simulink model "ssm_airframe_thrustvectored_test"  (R2022a)
settings: Solver=ode45  StartTime=0.0  StopTime=SimTime  RelTol=1e-3  AbsTol=1e-6
PreLoadFcn:
  | airframe_init
StopFcn:
  | airframe_plot
values from neighbouring files (symbols this model uses):
  ArmLength = 0.820 + 1.540    (= 2.36)    [airframe_init.m]
  boosting_time = 5    [airframe_init.m]
  thrust_magnitude = 78*1e+3    (= 78000)    [airframe_init.m]
undefined symbols (not defined in the file or in its folder): sigbuilder_block
libraries: shared6dof x1, simulink x1, simulink_extras x1
settings Model: Creator=amani  LastModifiedBy=amani

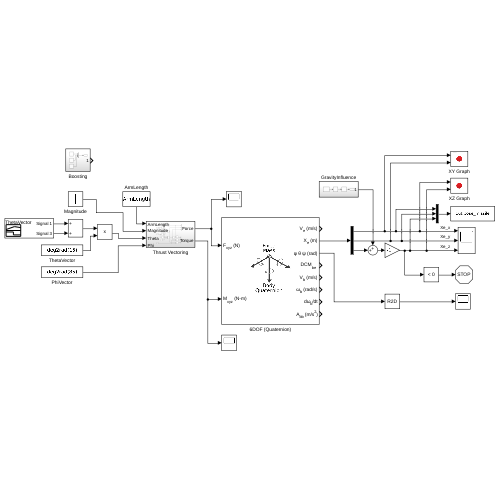
[thumbnail: Simulink's stored preview of the top-level diagram]
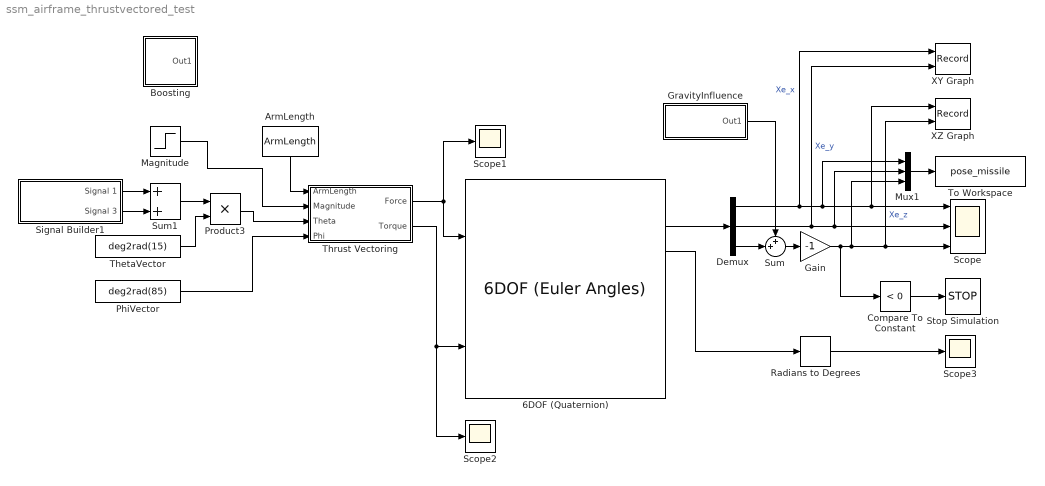
== system ssm_airframe_thrustvectored_test ==
  6DOF (Quaternion) : shared6dof/6DOF (Euler Angles)  units=Metric (MKS)  mtype=Fixed  rep=Quaternion  xme_0=pose_ini  Vm_0=vel_ini  eul_0=rot_ini  pm_0=rotvel_ini  mass_0=mass  mass_e=0.5  mass_f=2.0  inertia=inertia  inertia_e=eye(3)  inertia_f=2*eye(3)  k_quat=1.0  vre_flag=on  abi_flag=off  aMode=0  xme_statename=''  Vm_statename=''  eul_statename=''  quat_statename=''  pm_statename=''  mass_statename=''
      settings: SourceProductBaseCode=AE,PW,DR,MT,VE
  ArmLength : Constant  Value=ArmLength  VectorParams1D=off
  Boosting : Subsystem
  Compare To Constant : simulink/Logic and Bit Operations/Compare To Constant  relop=<  const=0  OutDataTypeStr=boolean
  Demux : Demux  Outputs=3
  Gain : Gain  Gain=-1
  GravityInfluence : Subsystem
  Magnitude : Step  Time=5  Before=thrust_magnitude  After=0  SampleTime=0
  Mux1 : Mux  Inputs=3
  PhiVector : Constant  Value=deg2rad(85)
  Product3 : Product
  Radians to Degrees : simulink_extras/Transformations/Radians to Degrees
  Scope : Scope  NumInputPorts=3
  Scope1 : Scope
  Scope2 : Scope
  Scope3 : Scope
  Signal Builder1 : Subsystem  Tag=STV Subsys  LoadFcn=sigbuilder_block('load');  StartFcn=sigbuilder_block('start');  StopFcn=sigbuilder_block('stop');  ClipboardFcn=sigbuilder_block('clipboard');  mask(Sigbuilder block){tuvar=[0:10]}
      mask help: Simulink:masks:SigbuilderBlock_MD
      mask init:
      | if ~strcmp(get_param(bdroot(gcbh),'SimulationStatus'),'stopped') tuvar = sigbuilder_block('maskInit'); end
      settings: CopyFcn=sigbuilder_block('copy');  DeleteFcn=sigbuilder_block('delete');  ModelCloseFcn=sigbuilder_block('modelClose');  PreSaveFcn=sigbuilder_block('preSave');  PauseFcn=sigbuilder_block('pause');  ContinueFcn=sigbuilder_block('continue');  NameChangeFcn=sigbuilder_block('namechange');  OpenFcn=sigbuilder_block('open',[40.5 0 1399.5 720.75 ]);  CloseFcn=sigbuilder_block('close');
      mask Display: plot(0, 0, 100, 100,[2, 2, 32, 32, 2], [68, 8, 8, 68, 68],[32, 2], [38, 38], [32, 19, 2],[53, 60, 44], [32, 17, 17, 2],[16, 16, 31, 31]);txt = getActiveGroup(gcbh);text(2, 100, txt,'verticalAlignment', 'top');
  Stop Simulation : Stop
  Sum : Sum  Inputs=++|
  Sum1 : Sum
  ThetaVector : Constant  Value=deg2rad(15)
  Thrust Vectoring : Subsystem
  To Workspace : ToWorkspace  VariableName=pose_missile  SaveFormat=Structure With Time  SampleTime=-1
  XY Graph : Record  FileSettingsInternal="{\"entries\":[{\"content\":{\"excelSettings\":{\"content\":{},\"type\":\"Streamout.ExcelSettings\"}},\"type\":\"Streamout.FileSettingStorage\",\"uuid\":\"0ebe5bd2-6dd8-4422-9468-a2e5212a589c\"}],\"packageUris\":[\"http://schema.mathworks.com/mf0/streamout_blocks/R2020a\"],\"version\":\"1.0\"}"  Layout=[1 1]  SignalsInternal="{\"entries\":[{\"content\":{\"signals\":[{\"content\":{\"blockPath\":[\"ssm_airframe_thrustvectored_test/XY Graph\"],\"channel\":[],\"dimensions\":[1],\"domain\":\"ssm_airframe_thrustvectored_test/XY Graph\",\"lineColor\":\"#a2142f\",\"plots\":[1],\"port\":1,\"sid\":[\"\"],\"signalID\":2033,\"signalName\":\"Xe_x\"},\"type\":\"RecordBlkView.Signal\",\"uuid\":\"929725db-a9ff-4e40-934e-6f60430dcc31\"},{\"content\":{\"blockPath\":[\"ssm_airframe_thrustvectored_test/XY Graph\"],\"channel\":[],\"dimensions\":[1],\"domain\":\"ssm_airframe_thrustvectored_test/XY Graph\",\"lineColor\":\"#139fff\",\"plots\":[1],\"port\":2,\"sid\":[\"\"],\"signalID\":2037,\"signalName\":\"Xe_y\"},\"type\":\"RecordBlkView.Signal\",\"uuid\":\"1de2dc4e-5c32-4d5d-ac98-cd5ddb664dcb\"}]},\"type\":\"RecordBlkView.InputSignals\",\"uuid\":\"a82f1b7b-1438-4de9-aa00-4fe59ea993c8\"}],\"packageUris\":[\"http://schema.mathworks.com/mf0/streamout_blocks/R2020a\"],\"version\":\"1.0\"}"  VisualizationBindings="{\"xyplotplugin\":{\"info\":[{\"series\":[{\"bindingParametersList\":[{\"parameter\":\"X-Axis\",\"signalID\":2033,\"signalName\":\"Xe_x\"},{\"parameter\":\"Y-Axis\",\"signalID\":2037,\"signalName\":\"Xe_y\"}],\"seriesID\":26156}],\"subplotID\":1}]}}"  CompatibilityTag=XY
  XZ Graph : Record  FileSettingsInternal="{\"entries\":[{\"content\":{\"excelSettings\":{\"content\":{},\"type\":\"Streamout.ExcelSettings\"}},\"type\":\"Streamout.FileSettingStorage\",\"uuid\":\"bbd1cac7-7029-4a9d-b9ac-d55883903ed7\"}],\"packageUris\":[\"http://schema.mathworks.com/mf0/streamout_blocks/R2020a\"],\"version\":\"1.0\"}"  Layout=[1 1]  SignalsInternal="{\"entries\":[{\"content\":{\"signals\":[{\"content\":{\"blockPath\":[\"ssm_airframe_thrustvectored_test/XZ Graph\"],\"channel\":[],\"dimensions\":[1],\"domain\":\"ssm_airframe_thrustvectored_test/XZ Graph\",\"lineColor\":\"#a2142f\",\"plots\":[1],\"port\":1,\"sid\":[\"\"],\"signalID\":2041,\"signalName\":\"Xe_x\"},\"type\":\"RecordBlkView.Signal\",\"uuid\":\"0a9b8eae-95df-4890-bdce-3116e9e64470\"},{\"content\":{\"blockPath\":[\"ssm_airframe_thrustvectored_test/XZ Graph\"],\"channel\":[],\"dimensions\":[1],\"domain\":\"ssm_airframe_thrustvectored_test/XZ Graph\",\"lineColor\":\"#139fff\",\"plots\":[1],\"port\":2,\"sid\":[\"\"],\"signalID\":2045,\"signalName\":\"Xe_z\"},\"type\":\"RecordBlkView.Signal\",\"uuid\":\"3959e62f-dd22-4433-954b-9d04f4581c5f\"}]},\"type\":\"RecordBlkView.InputSignals\",\"uuid\":\"aa5ce69c-9ff5-428d-bb5e-9516fd4365a3\"}],\"packageUris\":[\"http://schema.mathworks.com/mf0/streamout_blocks/R2020a\"],\"version\":\"1.0\"}"  VisualizationBindings="{\"xyplotplugin\":{\"info\":[{\"series\":[{\"bindingParametersList\":[{\"parameter\":\"X-Axis\",\"signalID\":2041,\"signalName\":\"Xe_x\"},{\"parameter\":\"Y-Axis\",\"signalID\":2045,\"signalName\":\"Xe_z\"}],\"seriesID\":25179}],\"subplotID\":1}]}}"  CompatibilityTag=XY
  wires:
  6DOF (Quaternion)/2 -> Demux/1
  Gain/1 -> XZ Graph/2, Scope/3, Mux1/3, Compare To Constant/1  "Xe_z"
  Sum/1 -> Gain/1
  Compare To Constant/1 -> Stop Simulation/1
  Demux/2 -> XY Graph/2, Scope/2, Mux1/2  "Xe_y"
  Demux/1 -> XY Graph/1, XZ Graph/1, Scope/1, Mux1/1  "Xe_x"
  Mux1/1 -> To Workspace/1
  GravityInfluence/1(Out1) -> Sum/1
  Demux/3 -> Sum/2
  Signal Builder1/1(Signal 1) -> Sum1/1
  Sum1/1 -> Product3/1
  ThetaVector/1 -> Product3/2
  Magnitude/1 -> Thrust Vectoring/2(Magnitude)
  Product3/1 -> Thrust Vectoring/3(Theta)
  PhiVector/1 -> Thrust Vectoring/4(Phi)
  Thrust Vectoring/1(Force) -> 6DOF (Quaternion)/1, Scope1/1
  ArmLength/1 -> Thrust Vectoring/1(ArmLength)
  Signal Builder1/2(Signal 3) -> Sum1/2
  6DOF (Quaternion)/3 -> Radians to Degrees/1
  Radians to Degrees/1 -> Scope3/1
  Thrust Vectoring/2(Torque) -> 6DOF (Quaternion)/2, Scope2/1

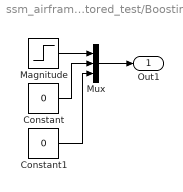
== system ssm_airframe_thrustvectored_test/Boosting ==
  Constant : Constant  Value=0
  Constant1 : Constant  Value=0
  Magnitude : Step  Time=boosting_time  Before=thrust_magnitude  After=0  SampleTime=0
  Mux : Mux  Inputs=3
  Out1 : Outport
  wires:
  Constant/1 -> Mux/2
  Constant1/1 -> Mux/3
  Magnitude/1 -> Mux/1
  Mux/1 -> Out1/1

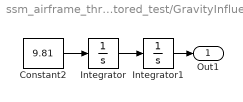
== system ssm_airframe_thrustvectored_test/GravityInfluence ==
  Constant2 : Constant  Value=9.81
  Integrator : Integrator
  Integrator1 : Integrator
  Out1 : Outport
  wires:
  Integrator/1 -> Integrator1/1
  Constant2/1 -> Integrator/1
  Integrator1/1 -> Out1/1

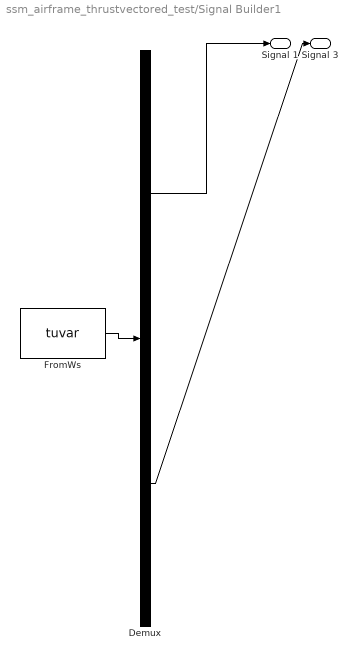
== system ssm_airframe_thrustvectored_test/Signal Builder1 ==
  Demux : Demux  Tag=STV Demux  Outputs=2
      settings: DisplayOption=none
  FromWs : FromWorkspace  Tag=STV FromWs  VariableName=tuvar
      SigBuilderData=|
      | common.afterFinalStr = 'Extrapolate'
      | common.sampleTime = 0
      | dataSet.timeRange = [0 60]
      | dataSet.name = 'ThetaVector'
      | sbobj.Groups.Name = 'ThetaVector'
      | sbobj.Groups.Signals(1).Name = 'Signal 1'
      | sbobj.Groups.Signals(1).XData = [0 1 2 3 60]
      | sbobj.Groups.Signals(1).YData = [0 0 1 0 0]
      | sbobj.Groups.Signals(2).Name = 'Signal 3'
      | sbobj.Groups.Signals(2).XData = [0 3 4 5 60]
      | sbobj.Groups.Signals(2).YData = [0 0 -2 0 0]
      | sbobj.Groups.TimeRange = [0 60]
  Signal 1 : Outport  Tag=STV Outport
  Signal 3 : Outport  Tag=STV Outport  Port=2
  wires:
  FromWs/1 -> Demux/1
  Demux/1 -> Signal 1/1
  Demux/2 -> Signal 3/1

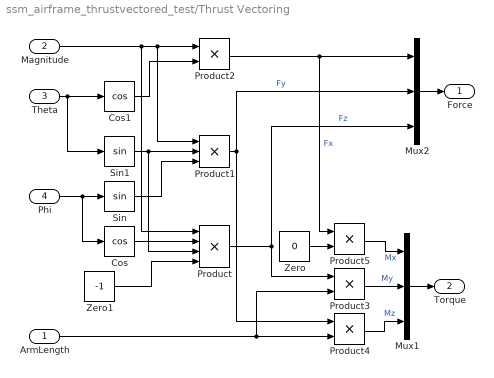
== system ssm_airframe_thrustvectored_test/Thrust Vectoring ==
  ArmLength : Inport
  Magnitude : Inport  Port=2
  Theta : Inport  Port=3
  Phi : Inport  Port=4
  Cos : Trigonometry  Operator=cos
  Cos1 : Trigonometry  Operator=cos
  Mux1 : Mux  Inputs=3
  Mux2 : Mux  Inputs=3
  Product : Product  Inputs=4
  Product1 : Product  Inputs=3
  Product{2..5} (4 alike) : Product
  Sin : Trigonometry
  Sin1 : Trigonometry
  Zero : Constant  Value=0
  Zero1 : Constant  Value=-1
  Force : Outport
  Torque : Outport  Port=2
  wires:
  Product/1 -> Mux2/3, Product3/1  "Fz"
  Product1/1 -> Mux2/2, Product4/1  "Fy"
  Phi/1 -> Cos/1, Sin/1
  Sin1/1 -> Product/3, Product1/2
  Magnitude/1 -> Product1/1, Product2/1, Product/1
  Zero/1 -> Product5/2
  Product2/1 -> Product5/1, Mux2/1  "Fx"
  Cos1/1 -> Product2/2
  Product5/1 -> Mux1/1  "Mx"
  Sin/1 -> Product1/3
  Zero1/1 -> Product/4
  Cos/1 -> Product/2
  Mux2/1 -> Force/1
  Mux1/1 -> Torque/1
  ArmLength/1 -> Product4/2, Product3/2
  Theta/1 -> Cos1/1, Sin1/1
  Product4/1 -> Mux1/3  "Mz"
  Product3/1 -> Mux1/2  "My"
